simulink model "BusConcatenationDemo"  (Simulink 6.3)
settings: Solver=FixedStepDiscrete  StartTime=0.0  StopTime=10.0  FixedStep=1  RelTol=1e-3
InitFcn:
  | %% DSPBuilder Start
  | alt_dspbuilder_update_model(bdroot)
  | %% DSPBuilder End
libraries: allblocks_alteradspbuilder2 x9
settings Model: LastModifiedBy=delphick

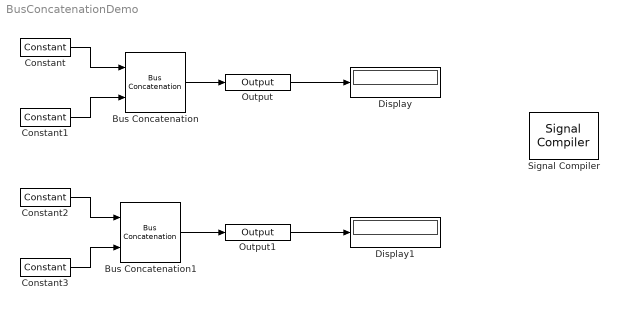
== system BusConcatenationDemo ==
  Bus Concatenation : allblocks_alteradspbuilder2/Bus Concatenation  isSigned=off  awidth=8  bwidth=2
  Bus Concatenation1 : allblocks_alteradspbuilder2/Bus Concatenation  isSigned=off  awidth=8  bwidth=2
  Constant : allblocks_alteradspbuilder2/Constant  mask_cst=73  BusType=Signed Integer  bwl=8  bwr=0  SpecifyClock=off
  Constant1 : allblocks_alteradspbuilder2/Constant  mask_cst=1  BusType=Signed Integer  bwl=2  bwr=0  SpecifyClock=off
  Constant2 : allblocks_alteradspbuilder2/Constant  mask_cst=73  BusType=Signed Integer  bwl=8  bwr=0  SpecifyClock=off
  Constant3 : allblocks_alteradspbuilder2/Constant  mask_cst=0  BusType=Signed Integer  bwl=2  bwr=0  SpecifyClock=off
  Display : Display
  Display1 : Display
  Output : allblocks_alteradspbuilder2/Output  iofile=C:\workspace_clean\Documentation\DesignExamples\Tutorials\UnitBlocks\IOBus\BusConcatenation\tb_BusConcatenationDemo\BusConcatenationDemo_Output.capture  BusType=Signed Integer  bwl=10  bwr=0  PORTTYPE=Output
  Output1 : allblocks_alteradspbuilder2/Output  iofile=C:\workspace_clean\Documentation\DesignExamples\Tutorials\UnitBlocks\IOBus\BusConcatenation\tb_BusConcatenationDemo\BusConcatenationDemo_Output1.capture  BusType=Signed Integer  bwl=10  bwr=0  PORTTYPE=Output
  Signal Compiler : allblocks_alteradspbuilder2/Signal Compiler  DeviceFamily=Stratix IV  DeviceName=AUTO  EnableSignalTap=off  SignalTapDepth=128  UseBoardBlock=off  StpUseDefaultClock=on  StpClock=clock
  wires:
  Constant/1 -> Bus Concatenation/1
  Constant1/1 -> Bus Concatenation/2
  Bus Concatenation/1 -> Output/1
  Constant2/1 -> Bus Concatenation1/1
  Constant3/1 -> Bus Concatenation1/2
  Bus Concatenation1/1 -> Output1/1
  Output1/1 -> Display1/1
  Output/1 -> Display/1
